simulink model "NR_30MHz_1carrier"  (R2022b)
settings: Solver=VariableStepAuto  StartTime=0.0  StopTime=0.05  RelTol=1e-3
undefined symbols (not defined in the file): waveform
settings Model: Creator=asmali  LastModifiedBy=asmali

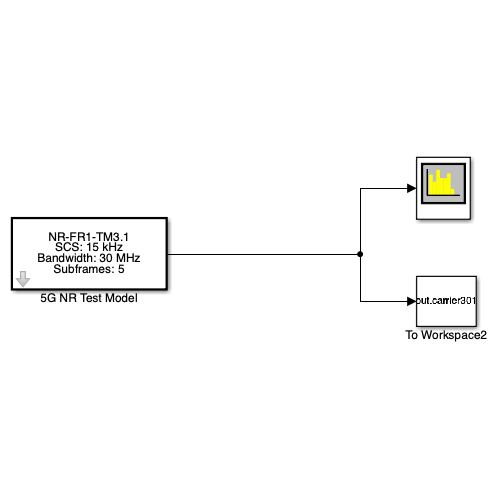
[thumbnail: Simulink's stored preview of the top-level diagram]
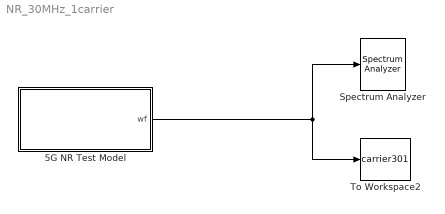
== system NR_30MHz_1carrier ==
  5G NR Test Model : MATLAB Function  Tag=BlockGeneratedWWGApp  TreatAsAtomicUnit=on  SystemSampleTime=1.6276041666666667447e-08  mask(5G NR Test Model Waveform Generator){nsamps=1, OutputAfterFinalValue=Cyclic repetition}
      mask prompts: nsamps "Samples per frame:"; OutputAfterFinalValue "Form output after final data value by:"
      mask init:
      | %% Generating NR Test Models waveform
      | % NR Test Models configuration
      | cfgDLTM = nrDLCarrierConfig;
      | cfgDLTM.Label = 'NR-FR1-TM3.1';
      | cfgDLTM.FrequencyRange = 'FR1';
      | cfgDLTM.ChannelBandwidth = 30;
      | cfgDLTM.NCellID = 1;
      | cfgDLTM.NumSubframes = 5;
      | cfgDLTM.WindowingPercent = 0;
      | cfgDLTM.SampleRate = [];
      | cfgDLTM.CarrierFrequency = 0;
      | 
      | %% SCS specific carriers
      | scscarrier = nrSCSCarrierConfig;
      | scscarrier.SubcarrierSpacing = 15;
      | scscarrier.NSizeGrid = 160;
      | scscarrier.NStartGrid = 0;
      | 
      | cfgDLTM.SCSCarriers = {scscarrier};
      | 
      | %% Bandwidth Parts
      | bwp = nrWavegenBWPConfig;
      | bwp.BandwidthPartID = 1;
      | bwp.Label = 'BWP1';
      | bwp.SubcarrierSpacing = 15;
      | bwp.CyclicPrefix = 'normal';
      | bwp.NSizeBWP = 160;
      | bwp.NStartBWP = 0;
      | 
      | cfgDLTM.BandwidthParts = {bwp};
      | 
      | %% Synchronization Signals Burst
      | ssburst = nrWavegenSSBurstConfig;
      | ssburst.Enable = false;
      | ssburst.Power = 0;
      | ssburst.BlockPattern = 'Case A';
      | ssburst.TransmittedBlocks = [1 0 0 0];
      | ssburst.Period = 10;
      | ssburst.NCRBSSB = [];
      | ssburst.KSSB = 0;
      | ssburst.DataSource = 'MIB';
      | ssburst.DMRSTypeAPosition = 2;
      | ssburst.CellBarred = false;
      | ssburst.IntraFreqReselection = false;
      | ssburst.PDCCHConfigSIB1 = 0;
      | ssburst.SubcarrierSpacingCommon = 30;
      | 
      | cfgDLTM.SSBurst = ssburst;
      | 
      | %% CORESET and Search Space Configuration
      | coreset = nrCORESETConfig;
      | coreset.CORESETID = 1;
      | coreset.Label = 'CORESET1';
      | coreset.FrequencyResources = 1;
      | coreset.Duration = 2;
      | coreset.CCEREGMapping = 'noninterleaved';
      | coreset.REGBundleSize = 2;
      | coreset.InterleaverSize = 2;
      | coreset.ShiftIndex = 0;
      | coreset.PrecoderGranularity = 'sameAsREG-bundle';
      | coreset.RBOffset = [];
      | 
      | cfgDLTM.CORESET = {coreset};
      | 
      | % Search Spaces
      | searchspace = nrSearchSpaceConfig;
      | searchspace.SearchSpaceID = 1;
      | searchspace.Label = 'SearchSpace1';
      | searchspace.CORESETID = 1;
      | searchspace.SearchSpaceType = 'common';
      | searchspace.StartSymbolWithinSlot = 0;
      | searchspace.SlotPeriodAndOffset = [1 0];
      | searchspace.Duration = 1;
      | searchspace.NumCandidates = [8 8 0 0 0];
      | 
      | cfgDLTM.SearchSpaces = {searchspace};
      | 
      | %% PDCCH Instances Configuration
      | pdcch = nrWavegenPDCCHConfig;
      | pdcch.Enable = true;
      | pdcch.Label = 'PDCCH1';
      | pdcch.Power = 0;
      | pdcch.BandwidthPartID = 1;
      | pdcch.SearchSpaceID = 1;
      | pdcch.AggregationLevel = 1;
      | pdcch.AllocatedCandidate = 1;
      | pdcch.CCEOffset = [];
      | pdcch.SlotAllocation = 0;
      | pdcch.Period = 1;
      | pdcch.Coding = false;
      | pdcch.DataBlockSize = 20;
      | pdcch.DataSource = 'PN23';
      | pdcch.RNTI = 0;
      | pdcch.DMRSScramblingID = 1;
      | pdcch.DMRSPower = 0;
      | 
      | cfgDLTM.PDCCH = {pdcch};
      | 
      | %% PDSCH Instances Configuration
      | % PDSCH 1
      | pdsch1 = nrWavegenPDSCHConfig;
      | pdsch1.Enable = true;
      | pdsch1.Label = 'Partial band PDSCH sequence with 64QAM modulation scheme (target, RNTI = 0)';
      | pdsch1.Power = 0;
      | pdsch1.BandwidthPartID = 1;
      | pdsch1.Modulation = '64QAM';
      | pdsch1.NumLayers = 1;
      | pdsch1.MappingType = 'A';
      | pdsch1.ReservedCORESET = [];
      | pdsch1.SymbolAllocation = [0 14];
      | pdsch1.SlotAllocation = 0;
      | pdsch1.Period = 1;
      | pdsch1.PRBSet = 3:159;
      | pdsch1.VRBToPRBInterleaving = 0;
      | pdsch1.VRBBundleSize = 2;
      | pdsch1.NID = [];
      | pdsch1.RNTI = 0;
      | pdsch1.Coding = false;
      | pdsch1.TargetCodeRate = 0.4785;
      | pdsch1.TBScaling = 1;
      | pdsch1.XOverhead = 0;
      | pdsch1.RVSequence = 0;
      | pdsch1.DataSource = 'PN23';
      | pdsch1.DMRSPower = 0;
      | pdsch1.EnablePTRS = false;
      | pdsch1.PTRSPower = 0;
      | 
      | % PDSCH Reserved PRB
      | pdsch1ReservedPRB = nrPDSCHReservedConfig;
      | pdsch1ReservedPRB.PRBSet = 0:2;
      | pdsch1ReservedPRB.SymbolSet = [0 1];
      | pdsch1ReservedPRB.Period = 1;
      | 
      | pdsch1.ReservedPRB = {pdsch1ReservedPRB};
      | 
      | % PDSCH DM-RS
      | pdsch1DMRS = nrPDSCHDMRSConfig;
      | pdsch1DMRS.DMRSConfigurationType = 1;
      | pdsch1DMRS.DMRSReferencePoint = 'CRB0';
      | pdsch1DMRS.DMRSTypeAPosition = 2;
      | pdsch1DMRS.DMRSAdditionalPosition = 1;
      | pdsch1DMRS.DMRSLength = 1;
      | pdsch1DMRS.CustomSymbolSet = [];
      | pdsch1DMRS.DMRSPortSet = [];
      | pdsch1DMRS.NIDNSCID = [];
      | pdsch1DMRS.NSCID = 0;
      | pdsch1DMRS.NumCDMGroupsWithoutData = 1;
      | pdsch1DMRS.DMRSDownlinkR16 = 0;
      | 
      | pdsch1.DMRS = pdsch1DMRS;
      | 
      | % PDSCH PT-RS
      | pdsch1PTRS = nrPDSCHPTRSConfig;
      | pdsch1PTRS.TimeDensity = 4;
      | pdsch1PTRS.FrequencyDensity = 2;
      | pdsch1PTRS.REOffset = '00';
      | pdsch1PTRS.PTRSPortSet = [];
      | 
      | pdsch1.PTRS = pdsch1PTRS;
      | 
      | % PDSCH 2
      | pdsch2 = nrWavegenPDSCHConfig;
      | pdsch2.Enable = true;
      | pdsch2.Label = 'Partial band PDSCH sequence with 64QAM modulation scheme (target, RNTI = 2)';
      | pdsch2.Power = 0;
      | pdsch2.BandwidthPartID = 1;
      | pdsch2.Modulation = '64QAM';
      | pdsch2.NumLayers = 1;
      | pdsch2.MappingType = 'A';
      | pdsch2.ReservedCORESET = [];
      | pdsch2.SymbolAllocation = [2 12];
      | pdsch2.SlotAllocation = 0;
      | pdsch2.Period = 1;
      | pdsch2.PRBSet = 0:2;
      | pdsch2.VRBToPRBInterleaving = 0;
      | pdsch2.VRBBundleSize = 2;
      | pdsch2.NID = [];
      | pdsch2.RNTI = 2;
      | pdsch2.Coding = false;
      | pdsch2.TargetCodeRate = 0.4785;
      | pdsch2.TBScaling = 1;
      | pdsch2.XOverhead = 0;
      | pdsch2.RVSequence = 0;
      | pdsch2.DataSource = 'PN23';
      | pdsch2.DMRSPower = 0;
      | pdsch2.EnablePTRS = false;
      | pdsch2.PTRSPower = 0;
      | 
      | pdschreserved = nrPDSCHReservedConfig;
      | pdschreserved.PRBSet = 0:2;
      | pdschreserved.SymbolSet = [0 1];
      | pdschreserved.Period = 1;
      | 
      | pdsch2.ReservedPRB = {pdschreserved};
      | 
      | pdschdmrs = nrPDSCHDMRSConfig;
      | pdschdmrs.DMRSConfigurationType = 1;
      | pdschdmrs.DMRSReferencePoint = 'CRB0';
      | pdschdmrs.DMRSTypeAPosition = 2;
      | pdschdmrs.DMRSAdditionalPosition = 1;
      | pdschdmrs.DMRSLength = 1;
      | pdschdmrs.CustomSymbolSet = [];
      | pdschdmrs.DMRSPortSet = [];
      | pdschdmrs.NIDNSCID = [];
      | pdschdmrs.NSCID = 0;
      | pdschdmrs.NumCDMGroupsWithoutData = 1;
      | pdschdmrs.DMRSDownlinkR16 = 0;
      | 
      | pdsch2.DMRS = pdschdmrs;
      | 
      | pdschptrs = nrPDSCHPTRSConfig;
      | pdschptrs.TimeDensity = 4;
      | pdschptrs.FrequencyDensity = 2;
      | pdschptrs.REOffset = '00';
      | pdschptrs.PTRSPortSet = [];
      | 
      | pdsch2.PTRS = pdschptrs;
      | 
      | cfgDLTM.PDSCH = {pdsch1,pdsch2};
      | 
      | %% CSI-RS Instances Configuration
      | csirs = nrWavegenCSIRSConfig;
      | csirs.Enable = false;
      | csirs.Label = 'CSIRS1';
      | csirs.Power = 0;
      | csirs.BandwidthPartID = 1;
      | csirs.CSIRSType = 'nzp';
      | csirs.CSIRSPeriod = 'on';
      | csirs.RowNumber = 1;
      | csirs.Density = 'three';
      | csirs.SymbolLocations = 0;
      | csirs.SubcarrierLocations = 0;
      | csirs.NumRB = 160;
      | csirs.RBOffset = 0;
      | csirs.NID = 1;
      | 
      | cfgDLTM.CSIRS = {csirs};
      | 
      | % Generation
      | [waveform,info] = nrWaveformGenerator(cfgDLTM);
      | 
      | Fs = info.ResourceGrids(1).Info.SampleRate; 								 % Specify the sample rate of the waveform in Hz
      | 
      | %% Configuring block: update parameters and UserData
      | % Get current block
      | thisBlock = gcb;
      | 
      | % Set info parameters
      | maskHandle = Simulink.Mask.get(thisBlock);
      | textFsDialog = maskHandle.getDialogControl('textFs');
      | textFsDialog.Prompt = ['Waveform sample rate (Fs): ' num2str(Fs*1e-6,'%.9g') ' MHz'];
      | textWfLengthDialog = maskHandle.getDialogControl('textWFLength');
      | textWfLengthDialog.Prompt = ['Waveform length: ' num2str(length(waveform)) ' samples'];
      | 
      | % Set sample time of the block
      | set_param(thisBlock, 'SystemSampleTime', num2str(nsamps/Fs,'%.20g'));
      | 
      | % Update UserData
      | outVar.WaveformConfig = cfgDLTM;
      | outVar.WaveformLength = length(waveform);
      | outVar.Fs = Fs;
      | set_param(thisBlock, 'UserData', outVar);
  Spectrum Analyzer : SpectrumAnalyzer
  To Workspace2 : ToWorkspace  VariableName=carrier301  SampleTime=-1
      settings: Save2DSignal=2-D array (concatenate along first dimension)
  wires:
  5G NR Test Model/1(wf) -> To Workspace2/1, Spectrum Analyzer/1

== matlab function NR_30MHz_1carrier/5G NR Test Model ==
  data: wf output; waveform parameter; nsamps parameter; OutputAfterFinalValue parameter
function wf = wfGenerator(waveform, nsamps, OutputAfterFinalValue)

% Create persistent variable
persistent src;

% Preallocate output
wf = complex(zeros(nsamps,size(waveform,2)));

if isempty(src)
    % Get action when signal ends
    if OutputAfterFinalValue == 1
        signalEndAction = 'Cyclic repetition';
    else
        signalEndAction = 'Set to zero';
    end
    
    % Initialize persistent dsp.SignalSource to get current frame
    src = dsp.SignalSource(waveform,nsamps,'SignalEndAction',signalEndAction);
end

% Extract current frame
wf(:,:) = src();

end
